simulink model "d5_b_1_model"  (R2025a)
settings: Solver=VariableStepAuto  StartTime=0.0  StopTime=10.0  RelTol=1e-3
undefined symbols (not defined in the file): A, B, Rd, Sd, Ts, Tsd
settings Model: Creator=Korisnik  LastModifiedBy=Korisnik

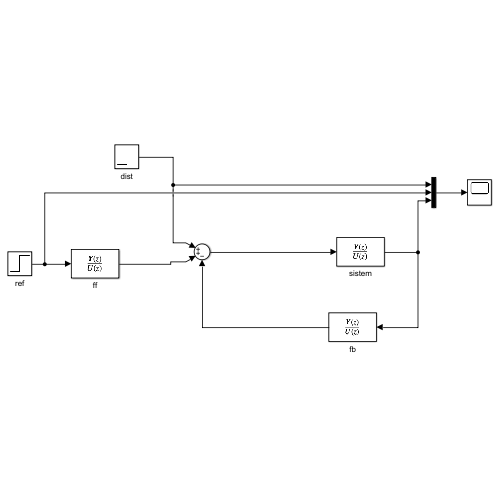
[thumbnail: Simulink's stored preview of the top-level diagram]
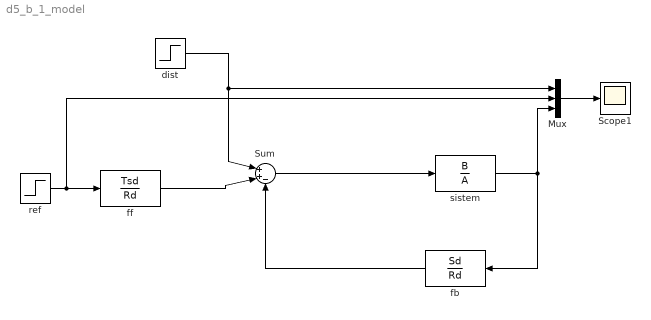
== system d5_b_1_model ==
  Mux : Mux  Inputs=3
  Scope1 : Scope
      settings: ActiveDisplayYMinimum=6.3574694230635149  ActiveDisplayYMaximum=8.6956101394269876
  Sum : Sum  Inputs=|++-
  dist : Step  Time=3  After=4  SampleTime=0
  fb : DiscreteTransferFcn  Numerator=Sd  Denominator=Rd
  ff : DiscreteTransferFcn  Numerator=Tsd  Denominator=Rd
  ref : Step  Time=0  After=8  SampleTime=Ts
  sistem : DiscreteTransferFcn  Numerator=B  Denominator=A
  wires:
  ref/1 -> Mux/2, ff/1
  sistem/1 -> Mux/3, fb/1
  ff/1 -> Sum/2
  dist/1 -> Sum/1, Mux/1
  fb/1 -> Sum/3
  Sum/1 -> sistem/1
  Mux/1 -> Scope1/1
